simulink model "untitled"  (R2022a)
settings: Solver=VariableStepAuto  StartTime=0.0  StopTime=10.0  RelTol=1e-3
settings Model: Creator=Waleed  LastModifiedBy=Waleed

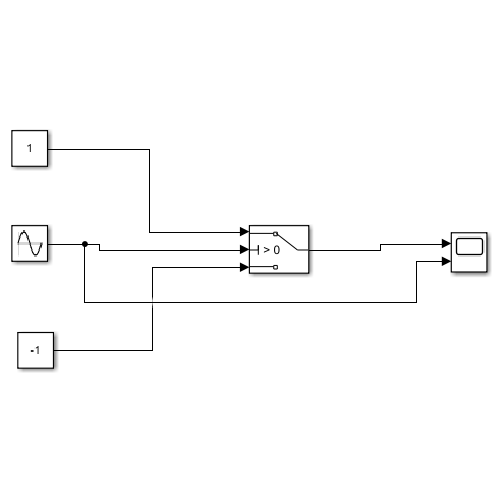
[thumbnail: Simulink's stored preview of the top-level diagram]
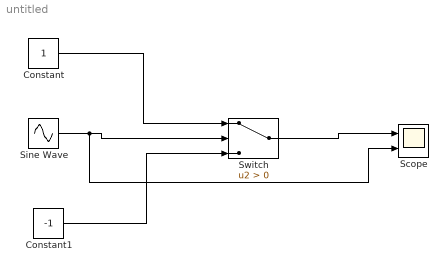
== system untitled ==
  Constant : Constant
  Constant1 : Constant  Value=-1
  Scope : Scope  NumInputPorts=2
  Sine Wave : Sin  SampleTime=0
  Switch : Switch  Criteria=u2 > Threshold  SaturateOnIntegerOverflow=off  InputSameDT=off
  wires:
  Constant1/1 -> Switch/3
  Constant/1 -> Switch/1
  Sine Wave/1 -> Scope/2, Switch/2
  Switch/1 -> Scope/1
